simulink library "TECSController"  (R2023a)
settings: Solver=VariableStepAuto  StartTime=0.0  StopTime=10.0  RelTol=1e-3
undefined symbols (not defined in the file): TECS, TO
libraries: simulink x10, simulink_extras x1, sharedtransform x1
settings Model: Creator=igmso  LastModifiedBy=igmso

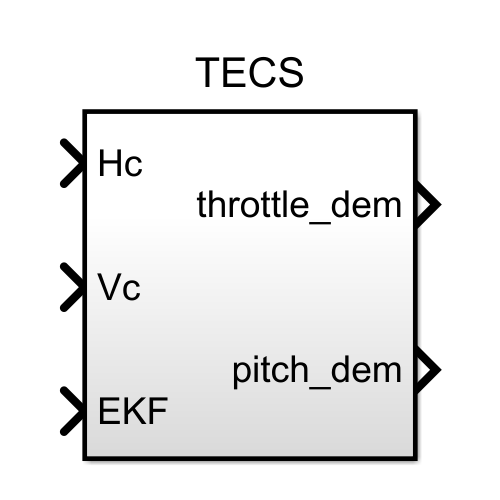
[thumbnail: Simulink's stored preview of the top-level diagram]
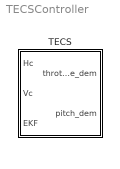
== system TECSController ==
  TECS : Subsystem  TreatAsAtomicUnit=on

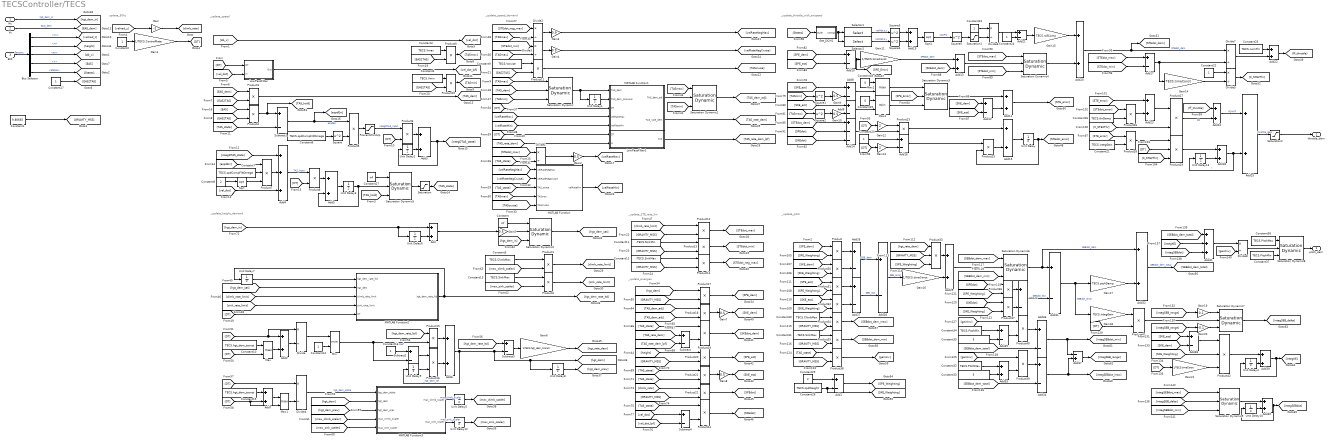
== system TECSController/TECS ==
  note: _update_energies
  note: update_50hz
  note: _update_speed
  note: _update_STE_rate_lim
  note: _update_speed_demand
  note: _update_height_demand
  note: _update_throttle_with_airspeed
  note: _update_pitch
  Hc : Inport  SampleTime=1/TECS.ControlRate
  Vc : Inport  Port=2  SampleTime=1/TECS.ControlRate
  EKF : Inport  Port=3  SampleTime=1/TECS.ControlRate
  Add{,2..3,5..7,11,15,18..20,22..25,29,32..33,39..40} (20 alike) : Sum
  Add{1,8..10,12,16..17,21,26..28,30..31,34..36,38} (17 alike) : Sum  Inputs=+-
  Add13 : Sum  Inputs=2
  Add14 : Sum  Inputs=+--
  Add37 : Sum  Inputs=-+
  Add4 : Sum  Inputs=3
  Add41 : Sum  Inputs=3
  Bus Selector : BusSelector  OutputSignals=Vz,H,ax,V,States
  Constant : Constant  Value=inf  SampleTime=1/TECS.ControlRate
  Constant1 : Constant  Value=9.80665  SampleTime=1/TECS.ControlRate
  Constant10 : Constant  Value=TECS.hgt_dem_tconst  SampleTime=1/TECS.ControlRate
  Constant11 : Constant  Value=-TECS.SinkMin  SampleTime=1/TECS.ControlRate
  Constant12 : Constant  Value=-TECS.SinkMax  SampleTime=1/TECS.ControlRate
  Constant13 : Constant  Value=TECS.SinkMax  SampleTime=1/TECS.ControlRate
  Constant{2,14,16..17,20,22..24} (8 alike) : Constant  SampleTime=1/TECS.ControlRate
  Constant15 : Constant  Value=TECS.hgt_dem_tconst  SampleTime=1/TECS.ControlRate
  Constant18 : Constant  Value=0  SampleTime=1/TECS.ControlRate
  Constant19 : Constant  Value=0  SampleTime=1/TECS.ControlRate
  Constant21 : Constant  Value=TECS.integGain  SampleTime=1/TECS.ControlRate
  Constant25 : Constant  Value=TECS.nomThr  SampleTime=1/TECS.ControlRate
  Constant26 : Constant  Value=TECS.thrDamp  SampleTime=1/TECS.ControlRate
  Constant27 : Constant  Value=inf  SampleTime=1/TECS.ControlRate
  Constant28 : Constant  Value=TECS.spdWeight  SampleTime=1/TECS.ControlRate
  Constant29 : Constant  Value=2  SampleTime=1/TECS.ControlRate
  Constant3 : Constant  Value=TECS.Vmax  SampleTime=1/TECS.ControlRate
  Constant30 : Constant  Value=TECS.ClimbMax  SampleTime=1/TECS.ControlRate
  Constant31 : Constant  Value=-TECS.SinkMax  SampleTime=1/TECS.ControlRate
  Constant32 : Constant  Value=TECS.PitchMax  SampleTime=1/TECS.ControlRate
  Constant33 : Constant  Value=5  SampleTime=1/TECS.ControlRate
  Constant34 : Constant  Value=TECS.PitchMin  SampleTime=1/TECS.ControlRate
  Constant35 : Constant  Value=5  SampleTime=1/TECS.ControlRate
  Constant36 : Constant  Value=TECS.PitchMax  SampleTime=1/TECS.ControlRate
  Constant37 : Constant  Value=TECS.PitchMin  SampleTime=1/TECS.ControlRate
  Constant4 : Constant  Value=TECS.Vmin  SampleTime=1/TECS.ControlRate
  Constant5 : Constant  Value=TECS.ClimbMax  SampleTime=1/TECS.ControlRate
  Constant6 : Constant  Value=TECS.spdCompFiltOmega  SampleTime=1/TECS.ControlRate
  Constant7 : Constant  Value=TECS.spdCompFiltOmega  SampleTime=1/TECS.ControlRate
  Constant8 : Constant  Value=2  SampleTime=1/TECS.ControlRate
  Constant9 : Constant  Value=TECS.Vcruise  SampleTime=1/TECS.ControlRate
  Divide{,1..8} (9 alike) : Product  Inputs=*/
  Gain : Gain  Gain=-1
  Gain1 : Gain  Gain=1/TECS.ControlRate
  Gain{2,5,7..10} (6 alike) : Gain  Gain=0.5
  Gain11 : Gain  Gain=1/TECS.timeConst
  Gain12 : Gain  Gain=2
  Gain13 : Gain  Gain=2
  Gain14 : Gain  Gain=TECS.timeConst
  Gain15 : Gain  Gain=TECS.rollComp
  Gain16 : Gain  Gain=1/TECS.timeConst
  Gain17 : Gain  Gain=TECS.ptchDamp
  Gain18 : Gain  Gain=TECS.integGain
  Gain19 : Gain  Gain=0.1
  Gain20 : Gain  Gain=-0.1
  Gain21 : Gain  Gain=1/TECS.timeConst
  Gain3 : Gain  Gain=0.9
  Gain4 : Gain  Gain=0.9
  Gain6 : Gain  Gain=1/TECS.hgt_dem_tconst
  Get_DCM1 : Subsystem
  LowPassFilter : Subsystem
  LowPassFilter1 : Subsystem
  MATLAB Function : MATLAB Function  TreatAsAtomicUnit=on
  MATLAB Function1 : MATLAB Function  TreatAsAtomicUnit=on
  MATLAB Function2 : MATLAB Function  TreatAsAtomicUnit=on
  MATLAB Function3 : MATLAB Function  TreatAsAtomicUnit=on
  Max : MinMax  Function=max  Inputs=2
  Max1 : MinMax  Function=max  Inputs=2
  Max2 : MinMax  Function=max  Inputs=2
  Max3 : MinMax  Inputs=2
  Min : MinMax  Inputs=2
  PreventWindUp : Saturate  UpperLimit=inf  LowerLimit=0
  Product{,1..6,8..28,30..32,34..41} (39 alike) : Product
  Product{7,29,33,42} (4 alike) : Product  Inputs=3
  Saturation : Saturate  UpperLimit=inf  LowerLimit=3
  Saturation Dynamic{,1..9} (10 alike) : simulink/Discontinuities/Saturation Dynamic  OutMin=[]  OutMax=[]  OutDataTypeStr=Inherit: Same as second input  OutDataType=fixdt(1, 16)  OutScaling=2^-10  DoSatur=off
  Saturation1 : Saturate  UpperLimit=1  LowerLimit=0.1
  Saturation2 : Saturate  UpperLimit=1  LowerLimit=0
  Selector1 : Selector  NumberOfDimensions=2  InputPortWidth=3  IndexOptions=Index vector (dialog),Index vector (dialog)  Indices=1,2  OutputSizes=1,1
  Selector2 : Selector  NumberOfDimensions=2  InputPortWidth=3  IndexOptions=Index vector (dialog),Index vector (dialog)  Indices=2,2  OutputSizes=1,1
  Sqrt : Sqrt
  Sqrt1 : Sqrt
  Square{,1..5} (6 alike) : Math  Operator=square
  Subtract{,1..4} (5 alike) : Sum  Inputs=+-
  Unit Delay : UnitDelay  SampleTime=1/TECS.ControlRate  StateName=STEdot_error  HasFrameUpgradeWarning=on
  Unit Delay1 : UnitDelay  SampleTime=1/TECS.ControlRate  StateName=TAS_dem_previous  HasFrameUpgradeWarning=on
  Unit Delay10 : UnitDelay  SampleTime=1/TECS.ControlRate  StateName=integSEBdot  HasFrameUpgradeWarning=on
  Unit Delay12 : UnitDelay  InitialCondition=1  SampleTime=1/TECS.ControlRate  StateName=max_sink_scaler  HasFrameUpgradeWarning=on
  Unit Delay13 : UnitDelay  SampleTime=1/TECS.ControlRate  StateName=integTHR_state  HasFrameUpgradeWarning=on
  Unit Delay2 : UnitDelay  SampleTime=1/TECS.ControlRate  StateName=integDTAS_state  HasFrameUpgradeWarning=on
  Unit Delay3 : UnitDelay  SampleTime=1/TECS.ControlRate  StateName=TAS_state  HasFrameUpgradeWarning=on
  Unit Delay4 : UnitDelay  SampleTime=1/TECS.ControlRate  StateName=integKE  HasFrameUpgradeWarning=on
  Unit Delay5 : UnitDelay  InitialCondition=1  SampleTime=1/TECS.ControlRate  StateName=max_climb_scaler  HasFrameUpgradeWarning=on
  Unit Delay6 : UnitDelay  InitialCondition=-TO.z  SampleTime=-1  StateName=hgt_dem_in_prev  HasFrameUpgradeWarning=on
  Unit Delay7 : UnitDelay  InitialCondition=-TO.z  SampleTime=1/TECS.ControlRate  StateName=hgt_dem_rate_ltd  HasFrameUpgradeWarning=on
  Unit Delay8 : UnitDelay  InitialCondition=-TO.z  SampleTime=1/TECS.ControlRate  StateName=hgt_dem_prev  HasFrameUpgradeWarning=on
  Unit Delay9 : UnitDelay  InitialCondition=-TO.z  SampleTime=1/TECS.ControlRate  StateName=hgt_dem_lpf  HasFrameUpgradeWarning=on
  throttle_dem : Outport  SampleTime=1/TECS.ControlRate
  pitch_dem : Outport  Port=2  SampleTime=1/TECS.ControlRate
  wires:
  Unit Delay10/1 -> Add40/2
  Unit Delay4/1 -> Add39/2
  Add40/1 -> [integSEBdot], Unit Delay10/1
  Saturation Dynamic9/1 -> Add40/1
  [integSEBdot_max] -> Saturation Dynamic9/1
  [integSEBdot_min] -> Saturation Dynamic9/3
  Constant36/1 -> Saturation Dynamic8/1
  Constant37/1 -> Saturation Dynamic8/3
  Divide8/1 -> Saturation Dynamic8/2
  [gainInv] -> Divide8/2
  Add41/1 -> Divide8/1
  [integKE] -> Add41/2
  [integSEBdot] -> Add41/3
  [SEBdot_dem_total] -> Add41/1
  [integSEB_delta] -> Saturation Dynamic9/2
  Add39/1 -> Unit Delay4/1, [integKE]
  Product42/1 -> Add39/1
  Gain21/1 -> Product42/3
  [DT] -> Gain21/1
  [SKE_Weighting] -> Product42/2
  Add38/1 -> Product42/1
  [SKE_dem] -> Add38/2
  [SKE_est] -> Add38/1
  Saturation Dynamic7/1 -> [integSEB_delta]
  Gain20/1 -> Saturation Dynamic7/3
  Gain19/1 -> Saturation Dynamic7/1
  Add37/1 -> [integSEB_range]
  [integSEB_range] -> Gain19/1
  [integSEB_range] -> Gain20/1
  Product41/1 -> Saturation Dynamic7/2
  [DT] -> Product41/2
  Gain18/1 -> Product41/1
  [gainInv] -> Product40/1
  Constant34/1 -> Add35/1
  Constant35/1 -> Add35/2
  Add35/1 -> Product40/2
  Product40/1 -> Add36/1
  [SEBdot_dem_total] -> Add36/2
  Add36/1 -> [integSEBdot_min], Add37/1
  Add34/1 -> [integSEBdot_max], Add37/2
  [SEBdot_dem_total] -> Add34/2
  Product39/1 -> Add34/1
  Add33/1 -> Product39/2
  Constant33/1 -> Add33/2
  Constant32/1 -> Add33/1
  [gainInv] -> Product39/1
  Product38/1 -> [gainInv]
  [GRAVITY_MSS] -> Product38/2
  [TAS_state] -> Product38/1
  Add32/1 -> [SEBdot_dem_total]  "SEBdot_dem_total"
  Gain17/1 -> Add32/2
  Add31/1 -> Gain17/1, Gain18/1  "SEBdot_error"
  Add30/1 -> Add31/2  "SEBdot_est"
  [SKEdot] -> Product37/1
  [SKE_Weighting] -> Product37/2
  [SPEdot] -> Product36/1
  [SPE_Weighting] -> Product36/2
  Product36/1 -> Add30/1
  Product37/1 -> Add30/2
  Saturation Dynamic6/1 -> Add31/1, Add32/1  "SEBdot_dem"
  Add29/1 -> Saturation Dynamic6/2
  [SEBdot_dem_max] -> Saturation Dynamic6/1
  [SEBdot_dem_min] -> Saturation Dynamic6/3
  Product35/1 -> [SEBdot_dem_min]
  Product34/1 -> [SEBdot_dem_max]
  Constant31/1 -> Product35/1
  [GRAVITY_MSS] -> Product35/2
  Constant30/1 -> Product34/1
  [GRAVITY_MSS] -> Product34/2
  Gain16/1 -> Add29/2
  Product33/1 -> Add29/1
  [SPE_Weighting] -> Product33/3
  [GRAVITY_MSS] -> Product33/2
  [hgt_rate_dem] -> Product33/1
  Add28/1 -> Gain16/1  "SEB_error"
  [SPE_est] -> Product31/1
  [SPE_Weighting] -> Product31/2
  [SKE_Weighting] -> Product32/2
  [SKE_est] -> Product32/1
  Product31/1 -> Add27/1
  Product32/1 -> Add27/2
  Add27/1 -> Add28/2  "SEB_est"
  Add26/1 -> Add28/1  "SEB_dem"
  Product30/1 -> Add26/2
  Product/1 -> Add26/1
  [SKE_dem] -> Product30/1
  [SKE_Weighting] -> Product30/2
  [SPE_Weighting] -> Product/2
  [SPE_dem] -> Product/1
  Add1/1 -> [SPE_Weighting]
  Constant28/1 -> Add1/2, [SKE_Weighting]
  Constant29/1 -> Add1/1
  Constant25/1 -> Add22/1
  Saturation Dynamic3/1 -> Add11/1
  [TAS_hold] -> Saturation Dynamic5/3
  Constant27/1 -> Saturation Dynamic5/1
  Saturation Dynamic5/1 -> Saturation/1
  Saturation Dynamic1/1 -> [TAS_dem_adj]
  Saturation2/1 -> throttle_dem/1
  Unit Delay1/1 -> MATLAB Function1/2(TAS_dem_previous)
  Add18/1 -> Add25/2, Unit Delay13/1  "I"
  Unit Delay13/1 -> Add18/2
  Product29/1 -> Add18/1
  [K_STE2Thr] -> Product29/3
  Product28/1 -> Product29/1
  [DT] -> Product29/2
  Constant21/1 -> Product28/2
  [STE_error] -> Product28/1
  Add24/1 -> Add25/1  "PD+FF"
  [ff_throttle] -> Add24/1
  Product27/1 -> Add24/2  "PD"
  [K_STE2Thr] -> Product27/2
  Add23/1 -> Product27/1
  Product26/1 -> Add23/2
  Constant26/1 -> Product26/2
  [STEdot_error] -> Product26/1
  [STE_error] -> Add23/1
  Add22/1 -> [ff_throttle]
  Divide7/1 -> Add22/2
  [STEdot_max] -> Add17/1
  [STEdot_min] -> Add17/2
  Gain14/1 -> Divide5/2
  Constant22/1 -> Divide5/1
  Divide5/1 -> [K_STE2Thr]
  Add17/1 -> Gain14/1, Divide7/2
  Gain15/1 -> Add20/1
  Constant24/1 -> Add21/2
  [States] -> Get_DCM1/1(Euler)
  Square5/1 -> Saturation1/1
  Divide6/1 -> Add21/1
  Square4/1 -> Add19/2
  Selector1/1 -> Square3/1  "rotMat.a.y"
  Add21/1 -> Gain15/1
  Selector2/1 -> Square4/1  "rotMat.b.y"
  Get_DCM1/1(rotMat) -> Selector1/1, Selector2/1
  Square3/1 -> Add19/1
  Constant23/1 -> Divide6/1
  Saturation1/1 -> Divide6/2
  Sqrt1/1 -> Square5/1  "cosPhi"
  Add19/1 -> Sqrt1/1
  Add20/1 -> Divide7/1, [STEdot_dem]  "STEdot_dem"
  Add15/1 -> Unit Delay/1
  Unit Delay/1 -> Product25/2, [STEdot_error]
  Product25/1 -> Add15/2
  Add16/1 -> Product25/1
  Constant20/1 -> Add16/1
  Gain13/1 -> Add16/2
  [DT] -> Gain13/1
  Product23/1 -> Add15/1
  Gain12/1 -> Product23/1
  [DT] -> Gain12/1
  Add14/1 -> Product23/2
  [SKEdot] -> Add14/3
  [SPEdot] -> Add14/2
  [STEdot_dem] -> Add14/1
  [STEdot_max] -> Saturation Dynamic4/1
  Add10/1 -> Gain11/1, [SPE_Error]
  [SKEdot_dem] -> Add13/2
  Gain11/1 -> Add13/1  "SPEdot_dem"
  Add13/1 -> Saturation Dynamic4/2
  [STEdot_min] -> Saturation Dynamic4/3
  [SPE_est] -> Add10/2
  Saturation Dynamic4/1 -> Add20/2
  [SPE_dem] -> Add10/1
  [SPE_Error] -> Saturation Dynamic3/2
  Add11/1 -> [STE_error]
  [SKE_dem] -> Add12/1
  [SKE_est] -> Add12/2
  Add12/1 -> Add11/2
  Max2/1 -> Saturation Dynamic3/1
  Max3/1 -> Saturation Dynamic3/3
  [TASmax] -> Square2/1
  Square2/1 -> Gain10/1
  Gain10/1 -> Add9/2
  [SKE_est] -> Add9/1
  Add9/1 -> Max3/2
  Constant19/1 -> Max3/1
  Constant18/1 -> Max2/1
  Add8/1 -> Max2/2
  [SKE_est] -> Add8/1
  Gain9/1 -> Add8/2
  Square1/1 -> Gain9/1
  [TASmin] -> Square1/1
  Constant17/1 -> [EAS2TAS]
  Product20/1 -> [SPE_est]
  Product22/1 -> [SPEdot]
  Product17/1 -> [SPE_dem]
  [TAS_state] -> Product21/1
  [TAS_rate_dem_lpf] -> Subtract/2
  [GRAVITY_MSS] -> Product20/2
  Subtract/1 -> Product19/2
  Gain8/1 -> [SKE_est]
  Product21/1 -> Gain8/1
  [height] -> Product20/1
  [vel_dot_lpf] -> Subtract4/2
  Subtract4/1 -> Product24/2
  [TAS_state] -> Product24/1
  Gain7/1 -> [SKE_dem]
  [TAS_dem_adj] -> Product18/2
  [TAS_dem_adj] -> Product18/1
  [climb_rate] -> Product22/1
  [TAS_state] -> Product19/1
  Product19/1 -> [SKEdot_dem]
  [GRAVITY_MSS] -> Product22/2
  [TAS_state] -> Product21/2
  Product18/1 -> Gain7/1
  [vel_dot] -> Subtract4/1
  Product24/1 -> [SKEdot]
  [hgt_dem] -> Product17/1
  [GRAVITY_MSS] -> Product17/2
  [TAS_rate_dem] -> Subtract/1
  [max_climb_scaler] -> Product1/2
  [max_sink_scaler] -> Product2/2
  MATLAB Function3/2(max_sink_scaler) -> Unit Delay12/1  "max_sink_scaler"
  MATLAB Function3/1(max_climb_scaler) -> Unit Delay5/1  "max_climb_scaler"
  [hgt_dem_prev] -> MATLAB Function3/3(hgt_dem_prev)
  Add7/1 -> Max1/1
  Max1/1 -> Divide4/2
  [max_climb_scaler] -> MATLAB Function3/4("max_climb_scaler ")
  [hgt_dem] -> MATLAB Function3/2(hgt_dem)
  [max_sink_scaler] -> MATLAB Function3/5("max_sink_scaler ")
  Divide4/1 -> MATLAB Function3/1(hgt_dem_alpha)  "hgt_dem_alpha"
  [DT] -> Divide4/1
  [DT] -> Add7/2, Max1/2
  Constant15/1 -> Add7/1
  Unit Delay8/1 -> [hgt_dem_prev]
  Gain6/1 -> [hgt_rate_dem]
  Subtract3/1 -> Gain6/1
  [hgt_dem_rate_ltd] -> Subtract3/1
  Add6/1 -> Unit Delay9/1, Subtract3/2, [hgt_dem], Unit Delay8/1  "_hgt_dem_lpf"
  Product16/1 -> Add6/2
  Unit Delay9/1 -> Product16/2
  Subtract2/1 -> Product16/1
  Constant16/1 -> Subtract2/1
  Product15/1 -> Add6/1
  Min/1 -> Product15/2, Subtract2/2  "coef"
  [hgt_dem_rate_ltd] -> Product15/1
  Divide/1 -> Min/1
  Constant14/1 -> Min/2
  Add2/1 -> Divide/2
  [DT] -> Add2/1, Divide/1
  Max/1 -> Add2/2
  [DT] -> Max/2
  Constant10/1 -> Max/1
  [DT] -> MATLAB Function2/5(DT)
  [sink_rate_limit] -> MATLAB Function2/4(sink_rate_limit)
  [climb_rate_limit] -> MATLAB Function2/3(climb_rate_limit)
  [hgt_dem_sat] -> MATLAB Function2/2(hgt_dem)
  MATLAB Function2/1(hgt_dem_rate_ltd) -> [hgt_dem_rate_ltd], Unit Delay7/1
  Unit Delay7/1 -> MATLAB Function2/1("hgt_dem_rate_ltd ")
  Constant/1 -> Saturation Dynamic2/1
  [hgt_dem_in] -> Saturation Dynamic2/3
  Saturation Dynamic2/1 -> [hgt_dem_sat]
  Gain5/1 -> Saturation Dynamic2/2
  Add/1 -> Gain5/1
  Unit Delay6/1 -> Add/2
  [hgt_dem_in] -> Unit Delay6/1, Add/1
  Product2/1 -> [sink_rate_limit]
  Constant13/1 -> Product2/1
  Product1/1 -> [climb_rate_limit]
  Constant5/1 -> Product1/1
  Saturation Dynamic/1 -> MATLAB Function1/1(TAS_dem), Unit Delay1/1
  [TASmax] -> Saturation Dynamic1/1
  [TASmin] -> Saturation Dynamic1/3
  MATLAB Function1/1(TAS_dem_adj) -> Saturation Dynamic1/2
  LowPassFilter1/1(Out) -> [TAS_rate_dem_lpf]
  [TAS_rate_dem] -> LowPassFilter1/2(In)
  MATLAB Function1/2(TAS_rate_dem) -> [TAS_rate_dem]
  [DT] -> LowPassFilter1/1(DT)
  [vel_dot] -> LowPassFilter/2(In)
  LowPassFilter/1(Out) -> [vel_dot_lpf]
  [DT] -> LowPassFilter/1(DT)
  [DT] -> MATLAB Function1/3(DT)
  [velRateMin] -> MATLAB Function1/5(velRateMin)
  [velRateMax] -> MATLAB Function1/4(velRateMax)
  [STEdot_min] -> Divide3/1
  Gain4/1 -> [velRateNegCruise]
  Divide3/1 -> Gain4/1
  [TASmax] -> Divide3/2
  MATLAB Function/1(velRateMin) -> [velRateMin]
  [TASmax] -> MATLAB Function/4(TASmax)
  [TAScruise] -> MATLAB Function/5(TAScruise)
  [velRateNegCruise] -> MATLAB Function/2(velRateNegCruise)
  [velRateNegMax] -> MATLAB Function/1(velRateNegMax)
  [TAS_state] -> MATLAB Function/3(TAS_state)
  [STEdot_neg_max] -> Divide2/1
  [TASmax] -> Divide2/2
  Divide2/1 -> Gain3/1
  Gain3/1 -> [velRateNegMax]
  Gain2/1 -> [velRateMax]
  Divide1/1 -> Gain2/1
  [TAS_state] -> Divide1/2
  [STEdot_max] -> Divide1/1
  Product14/1 -> [STEdot_neg_max]
  [GRAVITY_MSS] -> Product14/2
  Constant12/1 -> Product14/1
  Constant11/1 -> Product13/1
  [GRAVITY_MSS] -> Product13/2
  Product13/1 -> [STEdot_min]
  Product12/1 -> [STEdot_max]
  [GRAVITY_MSS] -> Product12/2
  [climb_rate_limit] -> Product12/1
  Product11/1 -> [TAScruise]
  [EAS2TAS] -> Product11/2
  Constant9/1 -> Product11/1
  Product10/1 -> [TASmin]
  [EAS2TAS] -> Product10/2
  Product9/1 -> [TASmax]
  [EAS2TAS] -> Product9/2
  [TAS_dem] -> Saturation Dynamic/2
  [TASmin] -> Saturation Dynamic/3
  [TASmax] -> Saturation Dynamic/1
  Saturation/1 -> [TAS_state]
  Add5/1 -> Unit Delay3/1
  Product8/1 -> Add5/1
  [DT] -> Product8/2
  Add4/1 -> Product8/1  "TAS_input"
  Product7/1 -> Add4/2
  [aspdErr] -> Product7/1
  Sqrt/1 -> Product7/3
  Constant7/1 -> Product7/2
  Constant8/1 -> Sqrt/1
  [vel_dot] -> Add4/3
  [integDTAS_state] -> Add4/1
  Add3/1 -> Unit Delay2/1, [integDTAS_state]
  Unit Delay2/1 -> Add3/2
  Product6/1 -> Add3/1
  [DT] -> Product6/2
  PreventWindUp/1 -> Product6/1  "integDTAS_input"
  Product5/1 -> PreventWindUp/1
  Square/1 -> Product5/2
  Constant6/1 -> Square/1
  Subtract1/1 -> Product5/1, [aspdErr]  "aspdErr"
  [TAS_state] -> Subtract1/2
  Product4/1 -> Subtract1/1, [TAS_hold]
  [EAS2TAS] -> Product4/2
  [EAS] -> Product4/1
  Product3/1 -> [TAS_dem]
  [EAS2TAS] -> Product3/2
  [EAS_dem] -> Product3/1
  [Ab_x] -> [vel_dot]
  Gain/1 -> [climb_rate]
  [velned_z] -> Gain/1
  Constant4/1 -> Product10/1
  Constant3/1 -> Product9/1
  Bus Selector/5 -> [States]  "<States>"
  Gain1/1 -> [DT]
  Constant2/1 -> Gain1/1
  Saturation Dynamic8/1 -> pitch_dem/1
  Add25/1 -> Saturation2/1  "throttle_dem"
  Bus Selector/4 -> [EAS]  "<V>"
  Bus Selector/3 -> [Ab_x]  "<ax>"
  Bus Selector/2 -> [height]  "<H>"
  Bus Selector/1 -> [velned_z]  "<Vz>"
  EKF/1 -> Bus Selector/1  "Sensors"
  Constant1/1 -> [GRAVITY_MSS]
  Vc/1 -> [EAS_dem]  "EAS_dem"
  Hc/1 -> [hgt_dem_in]  "hgt_dem_in"
  Unit Delay12/1 -> [max_sink_scaler]
  Unit Delay5/1 -> [max_climb_scaler]
  Unit Delay3/1 -> Add5/2, Saturation Dynamic5/2

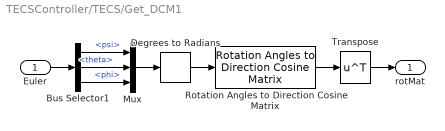
== system TECSController/TECS/Get_DCM1 ==
  Euler : Inport
  Bus Selector1 : BusSelector  OutputSignals=psi,theta,phi
  Degrees to Radians : simulink_extras/Transformations/Degrees to Radians
  Mux : Mux  Inputs=3
  Rotation Angles to Direction Cosine Matrix : sharedtransform/Rotation Angles to Direction Cosine Matrix  rotationOrder=ZYX  aMode=aMode
  Transpose : Math  Operator=transpose
  rotMat : Outport
  wires:
  Degrees to Radians/1 -> Rotation Angles to Direction Cosine Matrix/1
  Transpose/1 -> rotMat/1
  Bus Selector1/3 -> Mux/3  "<phi>"
  Bus Selector1/2 -> Mux/2  "<theta>"
  Euler/1 -> Bus Selector1/1
  Rotation Angles to Direction Cosine Matrix/1 -> Transpose/1
  Mux/1 -> Degrees to Radians/1
  Bus Selector1/1 -> Mux/1  "<psi>"

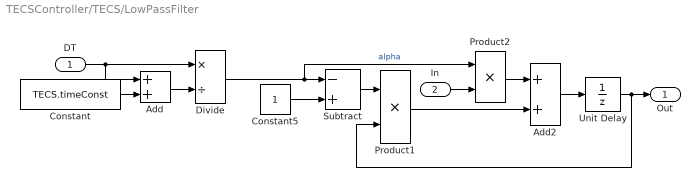
== system TECSController/TECS/LowPassFilter ==
  DT : Inport  SampleTime=1/TECS.ControlRate
  In : Inport  Port=2  SampleTime=1/TECS.ControlRate
  Add : Sum
  Add2 : Sum
  Constant : Constant  Value=TECS.timeConst  SampleTime=1/TECS.ControlRate
  Constant5 : Constant  SampleTime=1/TECS.ControlRate
  Divide : Product  Inputs=*/
  Product1 : Product
  Product2 : Product
  Subtract : Sum  Inputs=-+
  Unit Delay : UnitDelay  SampleTime=-1  StateName=vel_dot_lpf  HasFrameUpgradeWarning=on
  Out : Outport  SampleTime=1/TECS.ControlRate
  wires:
  In/1 -> Product2/2
  Add/1 -> Divide/2
  Unit Delay/1 -> Out/1, Product1/2
  Add2/1 -> Unit Delay/1
  Divide/1 -> Subtract/1, Product2/1  "alpha"
  Constant5/1 -> Subtract/2
  Constant/1 -> Add/2
  DT/1 -> Divide/1, Add/1
  Product1/1 -> Add2/2
  Product2/1 -> Add2/1
  Subtract/1 -> Product1/1

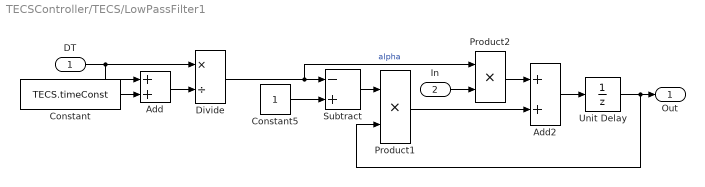
== system TECSController/TECS/LowPassFilter1 ==
  DT : Inport  SampleTime=1/TECS.ControlRate
  In : Inport  Port=2  SampleTime=1/TECS.ControlRate
  Add : Sum
  Add2 : Sum
  Constant : Constant  Value=TECS.timeConst  SampleTime=1/TECS.ControlRate
  Constant5 : Constant  SampleTime=1/TECS.ControlRate
  Divide : Product  Inputs=*/
  Product1 : Product
  Product2 : Product
  Subtract : Sum  Inputs=-+
  Unit Delay : UnitDelay  SampleTime=1/TECS.ControlRate  StateName={'TAS_rate_dem_lpf'}  HasFrameUpgradeWarning=on
  Out : Outport  SampleTime=1/TECS.ControlRate
  wires:
  In/1 -> Product2/2
  Add/1 -> Divide/2
  Unit Delay/1 -> Out/1, Product1/2
  Add2/1 -> Unit Delay/1
  Divide/1 -> Subtract/1, Product2/1  "alpha"
  Constant5/1 -> Subtract/2
  Constant/1 -> Add/2
  DT/1 -> Divide/1, Add/1
  Product1/1 -> Add2/2
  Product2/1 -> Add2/1
  Subtract/1 -> Product1/1

== matlab function TECSController/TECS/MATLAB Function1 ==
  data: TAS_dem input; TAS_dem_previous input; TAS_dem_adj output; DT input; velRateMax input; velRateMin input; TAS_rate_dem output
function [TAS_dem_adj, TAS_rate_dem] = apply_rate_limit(TAS_dem,TAS_dem_previous, DT, velRateMax, velRateMin)
if TAS_dem_previous == 0
    TAS_dem_previous = TAS_dem;
end
if ((TAS_dem - TAS_dem_previous) > (velRateMax * DT))
    TAS_dem_adj = TAS_dem_previous + velRateMax * DT;
    TAS_rate_dem = velRateMax;
elseif ((TAS_dem - TAS_dem_previous) < (velRateMin * DT))
    TAS_dem_adj = TAS_dem_previous + velRateMin * DT;
    TAS_rate_dem = velRateMin;
else
    TAS_rate_dem = (TAS_dem - TAS_dem_previous) / DT;
    TAS_dem_adj = TAS_dem;
end
end

== matlab function TECSController/TECS/MATLAB Function ==
  data: velRateNegMax input; velRateNegCruise input; TAS_state input; velRateMin output; TASmax input; TAScruise input
function velRateMin = velRateMin(velRateNegMax,velRateNegCruise,TAS_state,TASmax,TAScruise)
if velRateNegMax > velRateNegCruise
    % support either polarity
    temp = velRateNegMax;
    velRateNegMax = velRateNegCruise;
    velRateNegCruise = temp;
    temp = TASmax;
    TASmax = TAScruise;
    TAScruise = temp;
end
if TAS_state <= TASmax
    velRateMin = velRateNegMax;
elseif TAS_state >= TAScruise
    velRateMin = velRateNegCruise;
else
    p = (TAS_state - velRateNegMax) / (velRateNegCruise - velRateNegMax);
    velRateMin = TASmax + p * (TAScruise - TASmax);
end

== matlab function TECSController/TECS/MATLAB Function2 ==
  data: hgt_dem_rate_ltd input; hgt_dem input; hgt_dem_rate_ltd output; climb_rate_limit input; sink_rate_limit input; DT input
function hgt_dem_rate_ltd = limit_height_rate_of_change(hgt_dem_rate_ltd,hgt_dem, climb_rate_limit, sink_rate_limit, DT)
if ((hgt_dem - hgt_dem_rate_ltd) > (climb_rate_limit * DT))
    hgt_dem_rate_ltd = hgt_dem_rate_ltd + climb_rate_limit * DT;
elseif ((hgt_dem - hgt_dem_rate_ltd) < (-sink_rate_limit * DT))
    hgt_dem_rate_ltd = hgt_dem_rate_ltd - sink_rate_limit * DT;
else
    hgt_dem_rate_ltd = hgt_dem;
end
end

== matlab function TECSController/TECS/MATLAB Function3 ==
  data: hgt_dem_alpha input; max_climb_scaler output; hgt_dem input; hgt_dem_prev input; max_climb_scaler input; max_sink_scaler input; max_sink_scaler output
function [max_climb_scaler, max_sink_scaler] = update_scalers(hgt_dem_alpha, hgt_dem, hgt_dem_prev, max_climb_scaler, max_sink_scaler)
if (hgt_dem > hgt_dem_prev)
    max_climb_scaler = max_climb_scaler * (1.0 - hgt_dem_alpha);
elseif (hgt_dem < hgt_dem_prev)
    max_sink_scaler = max_sink_scaler * (1.0 - hgt_dem_alpha);
else
    max_climb_scaler = max_climb_scaler * (1.0 - hgt_dem_alpha) + hgt_dem_alpha;
    max_sink_scaler  =  max_sink_scaler * (1.0 - hgt_dem_alpha) + hgt_dem_alpha;
end
end
